simulink model "Measure_collection"  (R2021b)
settings: Solver=ode4  StartTime=0.0  StopTime=25  FixedStep=1e-2  RelTol=1e-3
values from neighbouring files (symbols this model uses):
  Ba = 0.02*ones(3,1)    [sensors_model.m]
  Bg = 5*ones(3,1)    [sensors_model.m]
settings Model: Creator=vince  LastModifiedBy=francescoiotti

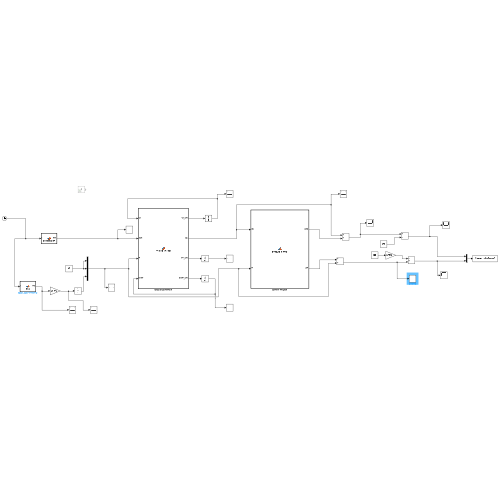
[thumbnail: Simulink's stored preview of the top-level diagram]
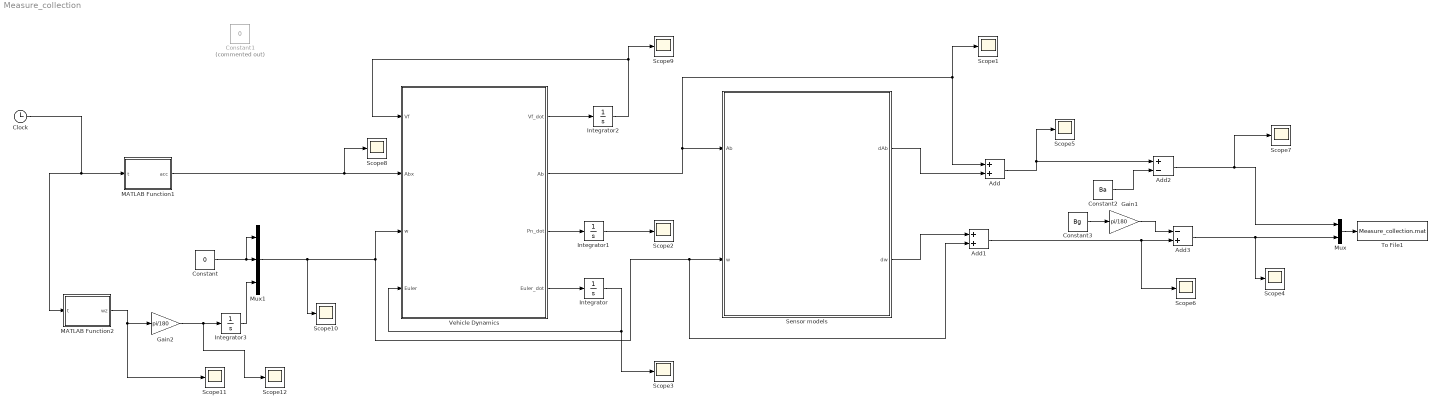
== system Measure_collection ==
  Add : Sum
  Add1 : Sum
  Add2 : Sum  Inputs=+-
  Add3 : Sum  Inputs=-+
  Clock : Clock
  Constant : Constant  Value=0
  Constant1 : Constant  Commented=on  Value=0
  Constant2 : Constant  Value=Ba
  Constant3 : Constant  Value=Bg
  Gain1 : Gain  Gain=pi/180
  Gain2 : Gain  Gain=pi/180
  Integrator : Integrator  InitialCondition=[0 0 0]'
  Integrator1 : Integrator  InitialCondition=[0 0 0]'
  Integrator2 : Integrator
  Integrator3 : Integrator
  MATLAB Function1 : MATLAB Function  TreatAsAtomicUnit=on
  MATLAB Function2 : MATLAB Function  TreatAsAtomicUnit=on
  Mux : Mux  Inputs=2
  Mux1 : Mux  Inputs=3
  Scope{1..12} (12 alike) : Scope
  Sensor models : MATLAB Function  TreatAsAtomicUnit=on
  To File1 : ToFile  Filename=Measure_collection.mat  MatrixName=measure
  Vehicle Dynamics : MATLAB Function  TreatAsAtomicUnit=on
  wires:
  Sensor models/1(dAb) -> Add/2
  Mux1/1 -> Scope10/1, Vehicle Dynamics/3(w), Add1/2, Sensor models/2(w)
  Sensor models/2(dw) -> Add1/1
  Add/1 -> Add2/1, Scope5/1
  Mux/1 -> To File1/1
  Vehicle Dynamics/4(Euler_dot) -> Integrator/1
  Vehicle Dynamics/3(Pn_dot) -> Integrator1/1
  Integrator/1 -> Scope3/1, Vehicle Dynamics/4(Euler)
  Integrator1/1 -> Scope2/1
  Add1/1 -> Scope6/1, Add3/2
  Vehicle Dynamics/2(Ab) -> Sensor models/1(Ab), Scope1/1, Add/1
  Vehicle Dynamics/1(Vf_dot) -> Integrator2/1
  Integrator2/1 -> Vehicle Dynamics/1(Vf), Scope9/1
  Constant2/1 -> Add2/2
  Add2/1 -> Scope7/1, Mux/1
  Add3/1 -> Scope4/1, Mux/2
  Constant3/1 -> Gain1/1
  Gain1/1 -> Add3/1
  Clock/1 -> MATLAB Function1/1(t), MATLAB Function2/1(t)
  MATLAB Function1/1(acc) -> Scope8/1, Vehicle Dynamics/2(Abx)
  Constant/1 -> Mux1/1, Mux1/2
  MATLAB Function2/1(wz) -> Gain2/1, Scope11/1
  Integrator3/1 -> Mux1/3
  Gain2/1 -> Scope12/1, Integrator3/1

== matlab function Measure_collection/Sensor models ==
  settings: updateMethod=DISCRETE
  data: Ab input; dAb output; w input; dw output
function [dAb, dw] = sensors_model(Ab, w)

%% Parameters

% Accelerometer
Ba = 0.02; % m/s^2
SFa = 0.05;
MISa = 0.1; % deg
stdv_a = 0.0055; % standard deviation
Wna = stdv_a*randn(3,1); % White Noise

Sa = [SFa MISa MISa;
      MISa SFa MISa;
      MISa MISa SFa];

% Gyros
Bg = 5*pi/180; % deg/s
SFg = 0;
MISg = 0.1*pi/180; % deg
stdv_g = 0.6325*pi/180; % standard deviation
Wng = stdv_g*randn(3,1); % White Noise

Sg = [SFg MISg MISg;
      MISg SFg MISg;
      MISg MISg SFg];

%% Models

% Accelerometer
dAb = Ba*ones(3,1) + Sa * Ab + Wna;

% Gyros
dw = Bg*ones(3,1) + Sg * w + Wng;

== matlab function Measure_collection/Vehicle Dynamics ==
  data: Vf input; Abx input; w input; Euler input; Vf_dot output; Ab output; Pn_dot output; Euler_dot output
function [Vf_dot, Ab, Pn_dot, Euler_dot] = Vehicle_model(Vf, Abx, w, Euler)
%% Land Vehicle Dynamic model
% x_dot is the derivative of x
wbx = w(1);
wby = w(2);
wbz = w(3);

% Euler angles
phi = Euler(1);
theta = Euler(2);
psi = Euler(3);

% Constant
g = 9.81;

% Model
Vf_dot = Abx - g*sin(theta);
Aby = Vf*wbz - g*sin(phi)*cos(theta);
Abz = -Vf*wby - g*cos(phi)*cos(theta);
phi_dot = wbx + sin(phi)*tan(theta)*wby + cos(phi)*tan(theta)*wbz;
theta_dot = cos(phi)*wby - sin(phi)*wbz;
psi_dot = sin(phi)/cos(theta)*wby + cos(phi)/cos(theta) * wbz;
Pnn_dot = Vf*cos(theta)*cos(psi);
Pne_dot = Vf*cos(theta)*sin(psi);
Pnd_dot = Vf*sin(theta);

Ab = [Abx, Aby, Abz]';
Euler_dot = [phi_dot, theta_dot, psi_dot]';
Pn_dot = [Pnn_dot, Pne_dot, Pnd_dot]';

== matlab function Measure_collection/MATLAB Function1 ==
  data: t input; acc output
function acc = acceleration(t)
% Parametri
% a = 10*pi^4;
Ka = 2.5;
Kd = -2.5;
c1 = 4;
c2 = 8;
c3 = 12;
c4 = 16;
c5 = 20;
c6 = 24;

% Accelerating part
if t < c2
    a = Ka * exp(-(t-c1)^2/2);

% Decelerating part
elseif t >= c2 && t < c3 
    a = Kd * exp(-(t-c3)^2/2);

% Inizio secondo picco di velocità
elseif t >= c3 && t < c4 
    a = 1.5 * exp(-(t-c3)^2/2);
% Decelero fino a fermarmi
elseif t >= c4 && t < c6 
    a = -2 * exp(-(t-c5)^2/2);
else
    a = 0;
end

acc = a;

== matlab function Measure_collection/MATLAB Function2 ==
  data: t input; wz output
function wz = ang(t)
% Parametri
% a = 10*pi^4;
Ka = 5;
Kd = -5;
c1 = 5;
c2 = 7.5;
c3 = 10;
c4 = 12.5;

% Accelerating part
if t < c1
    a = 0;
elseif t > c1 && t < c3
    a = Ka * exp(-(t-c2)^2/2);
% Decelerating part
% elseif t >= c1 && t < c2
%     a = Ka * exp(-(t-c2)^2/2);
% Decelerating part
elseif t >= c3 && t < 15 
    a = Kd * exp(-(t-c4)^2/2);
% Accelerating part
% elseif t >= c3 && t < c4
%     a = Kd * exp(-(t-c4)^2/2);
else
    a = 0;
end

wz= a;
